simulink model "Navigation_Full"  (R2016b)
settings: Solver=VariableStepAuto  StartTime=0.0  StopTime=10.0  RelTol=1e-3
values from neighbouring files (symbols this model uses):
  Env =     [UAV_modelconfig.mat]
undefined symbols (not defined in the file or in its folder): Earth, WGS84
libraries: Navigation_Lib x5, aerolibtransform2 x1
settings Model: Creator=UAVLAB  LastModifiedBy=UAVLAB

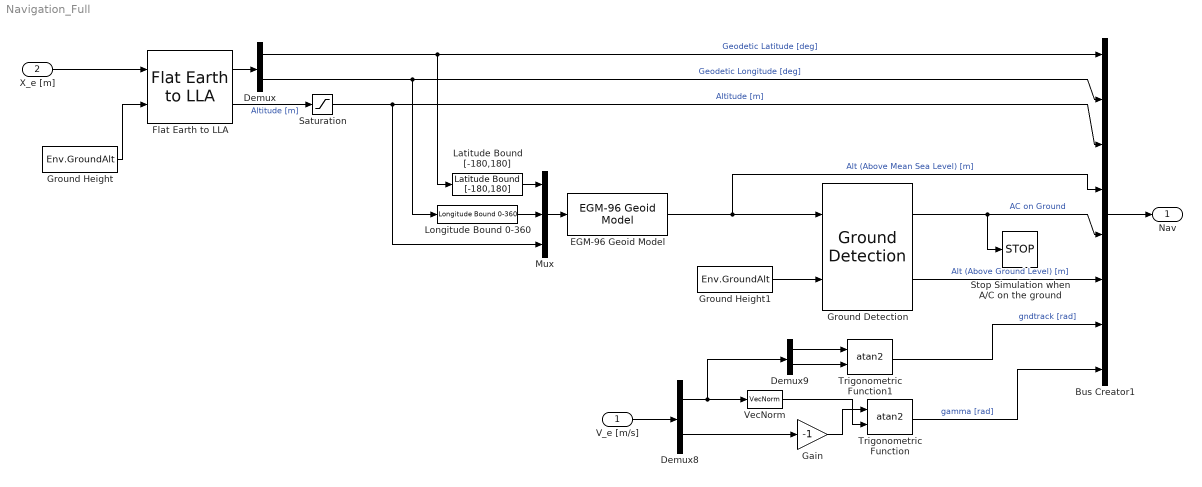
== system Navigation_Full ==
  V_e [m/s] : Inport
  X_e [m] : Inport  Port=2
  Bus Creator1 : BusCreator  Inputs=8  OutDataTypeStr=Bus: Nav
      settings: InheritFromInputs=off
  Demux : Demux  Outputs=2
  Demux8 : Demux  Outputs=[2 1]
  Demux9 : Demux  Outputs=2
  EGM-96 Geoid Model : Navigation_Lib/Navigation/EGM-96 Geoid Model
  Flat Earth to LLA : aerolibtransform2/Flat Earth to LLA  units=Metric (MKS)  ptype=Earth (WGS84)  F=1/298.257223563  R=6378137  LL0=TrimCondition.LLIni  psi=0
  Gain : Gain  Gain=-1
  Ground Detection : Navigation_Lib/Navigation/Ground Detection
  Ground Height : Constant  Value=Env.GroundAlt
  Ground Height1 : Constant  Value=Env.GroundAlt
  Latitude Bound [-180,180] : Navigation_Lib/Navigation/Latitude Bound [-180,180]
  Longitude Bound 0-360 : Navigation_Lib/Navigation/Longitude Bound 0-360
  Mux : Mux  Inputs=3
  Saturation : Saturate  UpperLimit=Inf  LowerLimit=0
  Stop Simulation when A/C on the ground : Stop
  Trigonometric Function : Trigonometry  Operator=atan2
  Trigonometric Function1 : Trigonometry  Operator=atan2
  VecNorm : Navigation_Lib/Navigation/VecNorm
  Nav : Outport  OutDataTypeStr=Bus: Nav
  wires:
  Flat Earth to LLA/1 -> Demux/1
  Flat Earth to LLA/2 -> Saturation/1  "Altitude [m]"
  Demux/1 -> Bus Creator1/1, Latitude Bound [-180,180]/1  "Geodetic Latitude [deg]"
  Demux/2 -> Bus Creator1/2, Longitude Bound 0-360/1  "Geodetic Longitude [deg]"
  X_e [m]/1 -> Flat Earth to LLA/1
  Ground Height/1 -> Flat Earth to LLA/2
  Bus Creator1/1 -> Nav/1
  EGM-96 Geoid Model/1 -> Ground Detection/1, Bus Creator1/4  "Alt (Above Mean Sea Level) [m]"
  Ground Height1/1 -> Ground Detection/2
  Ground Detection/1 -> Stop Simulation when A/C on the ground/1, Bus Creator1/5  "AC on Ground"
  Saturation/1 -> Bus Creator1/3, Mux/3  "Altitude [m]"
  Mux/1 -> EGM-96 Geoid Model/1
  Ground Detection/2 -> Bus Creator1/6  "Alt (Above Ground Level) [m]"
  V_e [m/s]/1 -> Demux8/1
  Demux8/2 -> Gain/1
  VecNorm/1 -> Trigonometric Function/2
  Trigonometric Function/1 -> Bus Creator1/8  "gamma [rad]"
  Demux9/2 -> Trigonometric Function1/2
  Trigonometric Function1/1 -> Bus Creator1/7  "gndtrack [rad]"
  Demux8/1 -> VecNorm/1, Demux9/1
  Demux9/1 -> Trigonometric Function1/1
  Longitude Bound 0-360/1 -> Mux/2
  Latitude Bound [-180,180]/1 -> Mux/1
  Gain/1 -> Trigonometric Function/1
